simulink model "PSDphaseTwoMark2"  (R2024b)
settings: Solver=VariableStepAuto  StartTime=0.0  StopTime=10.0  RelTol=1e-3
undefined symbols (not defined in the file or in its folder): Fs, N
libraries: dspstat3 x7, simulink x2, dspxfrm3 x2, dspsigops x2, eeGeneralControl x1
settings Model: Creator=potat  LastModifiedBy=potat

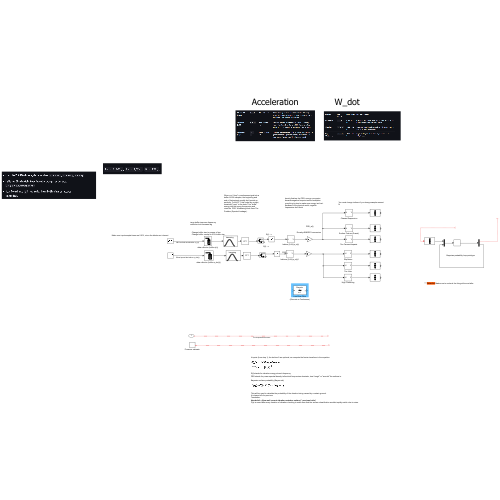
[thumbnail: Simulink's stored preview of the top-level diagram]
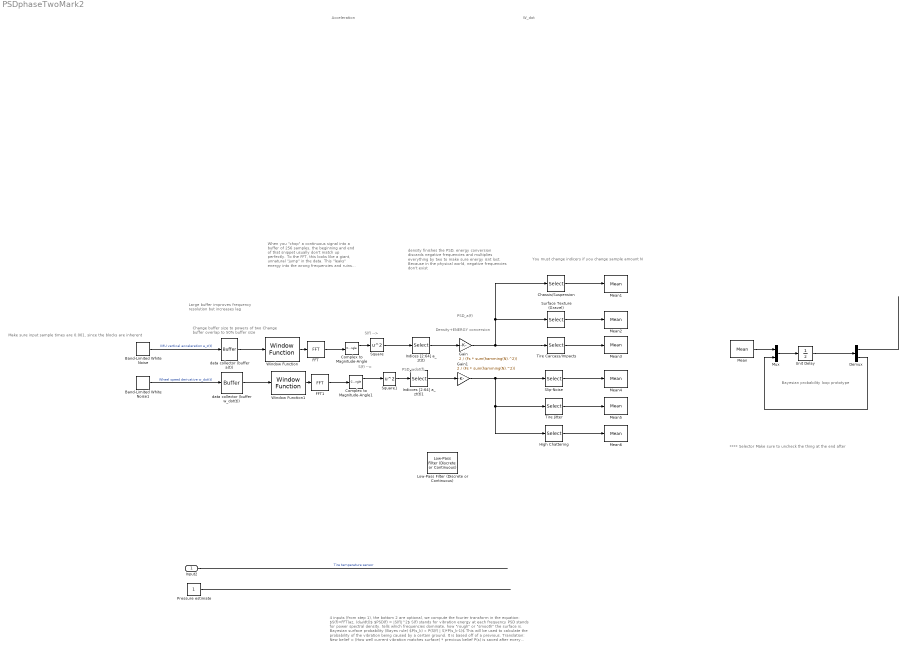
== system PSDphaseTwoMark2 ==
  note: Acceleration
  note: You must change indicers if you change sample amount
      | N
  note: density finishes the PSD, energy conversion discards negative frequencies and multiplies everything by two to make sure energy isnt lost. Because in the physical world, negative frequencies don't exist
  note: Density+ENERGY conversion
  note: Make sure input sample times are 0.001, since the blocks are inherent
  note: Bayesian probability loop prototype
  note: **** Selector Make sure to uncheck the thing at the end after
  note: When you "chop" a continuous signal into a buffer of 256 samples, the beginning and end of that snippet usually don't match up perfectly. To the FFT, this looks like a giant, unnatural "jump" in the data. This "leaks" energy into the wrong frequencies and ruins the PSD. Windowing block fixes The Problem (Spectral Leakage).
  note: Large buffer improves frequency resolution but increases lag
  note: Change buffer size to powers of two
      | Change buffer overlap to 50% buffer size
  note: S(f) -->
  note: 4 inputs (from step 1), the bottom 2 are optional, we compute the fourier transform in the equation:
      |
      | $S(f)=FFT(az​, (dω/dt))$
      | $PSD(f) = |S(f)|^2$
      |
      | S(f) stands for vibration energy at each frequency
      | PSD stands for power spectral density. tells which frequencies dominate, how "rough" or "smooth" the surface is.
      |
      | Bayesian surface probability (Bayes rule)
      |
      | $P(s_k) ∝ P(S(f) | S)*P(s_k-1)$
      |
      | This will be used to calculate the probability of the vibration being caused by a certain ground.
      | It is based off of a previous.
      | Translation:
      | New belief = (How well current vibration matches surface) * previous belief
      | P(s) is saved after every iteration of vibration checking to make sure that the surface classification wouldnt rapidly switch due to noise.
  note: S(f) -->
  note: PSD_a(f)
  note: PSD_wdot(f)
  note: W_dot
  Input2 : Inport
  Band-Limited White Noise : simulink/Sources/Band-Limited White Noise  Cov=[0.1]  Ts=0.001  seed=[23341]
  Band-Limited White Noise1 : simulink/Sources/Band-Limited White Noise  Cov=[0.1]  Ts=0.001  seed=[23341]
  Chassis/Suspension : Selector  IndexOptions=Index vector (dialog)  Indices=[1:3]  OutputSizes=1  RuntimeRangeChecks=on
  Complex to Magnitude-Angle : ComplexToMagnitudeAngle
  Complex to Magnitude-Angle1 : ComplexToMagnitudeAngle
  Demux : Demux  Outputs=2
  FFT : dspxfrm3/FFT  FFTImplementation=Auto  CompMethod=Table lookup  TableOpt=NEW  TableOptActive=Speed  BitRevOrder=off  Normalize=off  InheritFFTLength=on  FFTLength=128  WrapInput=on  roundingMode=Ceiling  overflowMode=off  firstCoeffDataTypeStr=Inherit: Same word length as input  firstCoeffLastDataTypeStr=Inherit: Same word length as input  outputMin=[]  outputMax=[]
  FFT1 : dspxfrm3/FFT  FFTImplementation=Auto  CompMethod=Table lookup  TableOpt=NEW  TableOptActive=Speed  BitRevOrder=off  Normalize=off  InheritFFTLength=on  FFTLength=64  WrapInput=on  roundingMode=Ceiling  overflowMode=off  firstCoeffDataTypeStr=Inherit: Same word length as input  firstCoeffLastDataTypeStr=Inherit: Same word length as input  outputMin=[]  outputMax=[]
  Gain : Gain  Gain=2 / (Fs * sum(hamming(N).^2))  OutMin=[1]  OutMax=[128]
  Gain1 : Gain  Gain=2 / (Fs * sum(hamming(N).^2))
  High Chattering : Selector  IndexOptions=Index vector (dialog)  Indices=[35:60]  OutputSizes=1  RuntimeRangeChecks=on
  Indicces [2:64] a_zt(t)1 : Selector  InputPortWidth=128  IndexOptions=Index vector (dialog)  Indices=[2:64]  OutputSizes=1  RuntimeRangeChecks=on
  Indices [2:64] a_zt(t) : Selector  InputPortWidth=128  IndexOptions=Index vector (dialog)  Indices=[2:64]  OutputSizes=1  RuntimeRangeChecks=on
  Low-Pass Filter (Discrete or Continuous) : eeGeneralControl/Low-Pass Filter (Discrete or Continuous)  K=1  T=1  B=inf  A=-inf  init_option=Inherited from block input  x0=0  Ts=-1
  Mean{,1..6} (7 alike) : dspstat3/Mean  run=off  InputProcessing=Columns as channels (frame based)  reset_popup=None  directionMode=Each column  dimension=1  roiEnable=off  roiType=Rectangles  roiPortion=Entire ROI  roiOutput=Individual statistics for each ROI  roiFlag=off  roundingMode=Floor  overflowMode=off  outputDataTypeStr=Inherit: Same as accumulator  outputMin=[]  outputMax=[]  outputLastDataTypeStr=Inherit: Same as accumulator
  Mux : Mux  Inputs=2
  Pressure estimate : Constant
  Slip-Noise : Selector  IndexOptions=Index vector (dialog)  Indices=[3:7]  OutputSizes=1  RuntimeRangeChecks=on
  Square : Math  Operator=square
  Square1 : Math  Operator=square
  Surface Texture (Gravel) : Selector  IndexOptions=Index vector (dialog)  Indices=[8:16]  OutputSizes=1  RuntimeRangeChecks=on
  "Tire Carcass/Impacts " : Selector  IndexOptions=Index vector (dialog)  Indices=[19:51]  OutputSizes=1  RuntimeRangeChecks=on
  Tire Jitter : Selector  IndexOptions=Index vector (dialog)  Indices=[13:25]  OutputSizes=1  RuntimeRangeChecks=on
  Unit Delay : UnitDelay  SampleTime=-1  HasFrameUpgradeWarning=on
  Window Function : dspsigops/Window Function  winmode=Apply window to input  wintype=Hamming  sampmode=Continuous  samptime=1  N=64  Rs=50  beta=10  winsamp=Symmetric  UserWindow=hamming  OptParams=off  UserParams={'symmetric'}  dataType=double  isSigned=on  wordLen=16  udDataType=sfix(16)  fracBitsMode=Best precision  numFracBits=15  roundingMode=Floor  overflowMode=off  numSidelobes=4  sidelobeLevel=-30
  Window Function1 : dspsigops/Window Function  winmode=Apply window to input  wintype=Hamming  sampmode=Continuous  samptime=1  N=64  Rs=50  beta=10  winsamp=Symmetric  UserWindow=hamming  OptParams=off  UserParams={'symmetric'}  dataType=double  isSigned=on  wordLen=16  udDataType=sfix(16)  fracBitsMode=Best precision  numFracBits=15  roundingMode=Floor  overflowMode=off  numSidelobes=4  sidelobeLevel=-30
  data collector (buffer a(t)) : Buffer  N=N  V=64  OutputFrames=off
  data collector (buffer w_dot(t)) : Buffer  N=128  V=64  OutputFrames=off
  wires:
  Band-Limited White Noise/1 -> data collector (buffer a(t))/1  "IMU vertical acceleration a_z(t)"
  Band-Limited White Noise1/1 -> data collector (buffer w_dot(t))/1  "Wheel speed derivative w_dot(t)"
  Input2/1 -> ?  "Tire temperature sensor"
  Pressure estimate/1 -> ?
  FFT/1 -> Complex to Magnitude-Angle/1
  data collector (buffer a(t))/1 -> Window Function/1
  Complex to Magnitude-Angle/1 -> Square/1
  data collector (buffer w_dot(t))/1 -> Window Function1/1
  FFT1/1 -> Complex to Magnitude-Angle1/1
  Complex to Magnitude-Angle1/1 -> Square1/1
  Square/1 -> Indices [2:64] a_zt(t)/1
  Window Function/1 -> FFT/1
  Window Function1/1 -> FFT1/1
  Square1/1 -> Indicces [2:64] a_zt(t)1/1
  Mean/1 -> Mux/1
  Unit Delay/1 -> Demux/1
  Demux/1 -> ?
  Demux/2 -> Mux/2
  Mux/1 -> Unit Delay/1
  Chassis/Suspension/1 -> Mean1/1
  Surface Texture (Gravel)/1 -> Mean2/1
  "Tire Carcass/Impacts "/1 -> Mean3/1
  Indicces [2:64] a_zt(t)1/1 -> Gain1/1
  Gain1/1 -> High Chattering/1, Tire Jitter/1, Slip-Noise/1
  Slip-Noise/1 -> Mean4/1
  Tire Jitter/1 -> Mean5/1
  High Chattering/1 -> Mean6/1
  ? -> Mean/1
  Indices [2:64] a_zt(t)/1 -> Gain/1
  Gain/1 -> "Tire Carcass/Impacts "/1, Surface Texture (Gravel)/1, Chassis/Suspension/1
